simulink model "simula_LPV_RST_2D0F"  (R2017a)
settings: Solver=VariableStepAuto  StartTime=0.0  StopTime=tsim  RelTol=1e-3
values from neighbouring files (symbols this model uses):
  Am = CL_Perf(Tr,MaxOvershoot,Ts)    [Principal_LPV_RST_2DOF.m]
  Asim = double(A_LPV)    [Principal_LPV_RST_2DOF.m]
  Bm = [sum(Am)]    [Principal_LPV_RST_2DOF.m]
  Bsim = double([zeros(1,d) B_LPV])    [Principal_LPV_RST_2DOF.m]
  KTsim = 1/KTsim    [Principal_LPV_RST_2DOF.m]
  Rsim = double(R_LPV)    [Principal_LPV_RST_2DOF.m]
  Ssim = double(S_LPV)    [Principal_LPV_RST_2DOF.m]
  Ts = 0.05    [Principal_LPV_RST_2DOF.m]
  Tsim = double(T_LPV)    [Principal_LPV_RST_2DOF.m]
settings Model: Creator=FABRICIO  LastModifiedBy=Fabricio

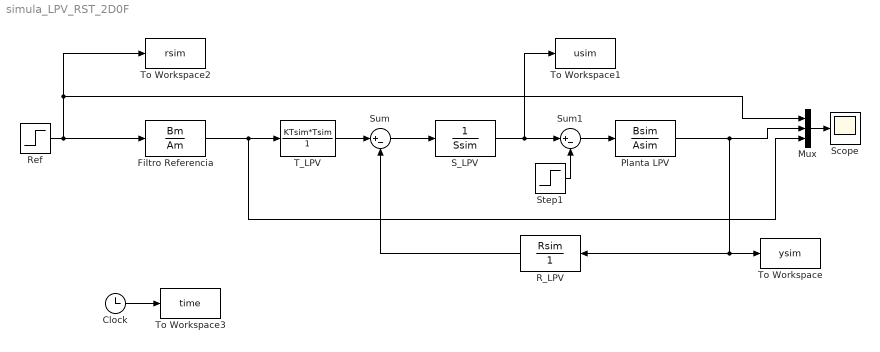
== system simula_LPV_RST_2D0F ==
  Clock : Clock
  Filtro Referencia : DiscreteFilter  Numerator=Bm  Denominator=Am  SampleTime=Ts
  Mux : Mux  Inputs=3
  Planta LPV : DiscreteFilter  Numerator=Bsim  Denominator=Asim  SampleTime=Ts
  R_LPV : DiscreteFilter  Numerator=Rsim  Denominator=1  SampleTime=Ts
  Ref : Step  SampleTime=0
  S_LPV : DiscreteFilter  Numerator=1  Denominator=Ssim  SampleTime=Ts
  Scope : Scope
  Step1 : Step  Time=4  After=0.1  SampleTime=0
  Sum : Sum  Inputs=|+-
  Sum1 : Sum  Inputs=|+-
  T_LPV : DiscreteFilter  Numerator=KTsim*Tsim  Denominator=1  SampleTime=Ts
  To Workspace : ToWorkspace  VariableName=ysim  SampleTime=Ts
  To Workspace1 : ToWorkspace  VariableName=usim  SampleTime=Ts
  To Workspace2 : ToWorkspace  VariableName=rsim  SampleTime=Ts
  To Workspace3 : ToWorkspace  VariableName=time  SampleTime=Ts
  wires:
  Sum/1 -> S_LPV/1
  R_LPV/1 -> Sum/2
  Mux/1 -> Scope/1
  T_LPV/1 -> Sum/1
  Clock/1 -> To Workspace3/1
  S_LPV/1 -> To Workspace1/1, Sum1/1
  Step1/1 -> Sum1/2
  Planta LPV/1 -> Mux/2, To Workspace/1, R_LPV/1
  Ref/1 -> Filtro Referencia/1, Mux/1, To Workspace2/1
  Filtro Referencia/1 -> T_LPV/1, Mux/3
  Sum1/1 -> Planta LPV/1
